simulink model "twolvl_test"  (Simulink 7.5)
settings: Solver=ode45  StartTime=0.0  StopTime=0.5  RelTol=1e-3
undefined symbols (not defined in the file or in its folder): D1, Delta, Ts
libraries: powerlib x18, powerlib_extras x1
settings Model: Creator=IS  LastModifiedBy=IS
settings SolverCC: ZeroCrossAlgorithm=Adaptive

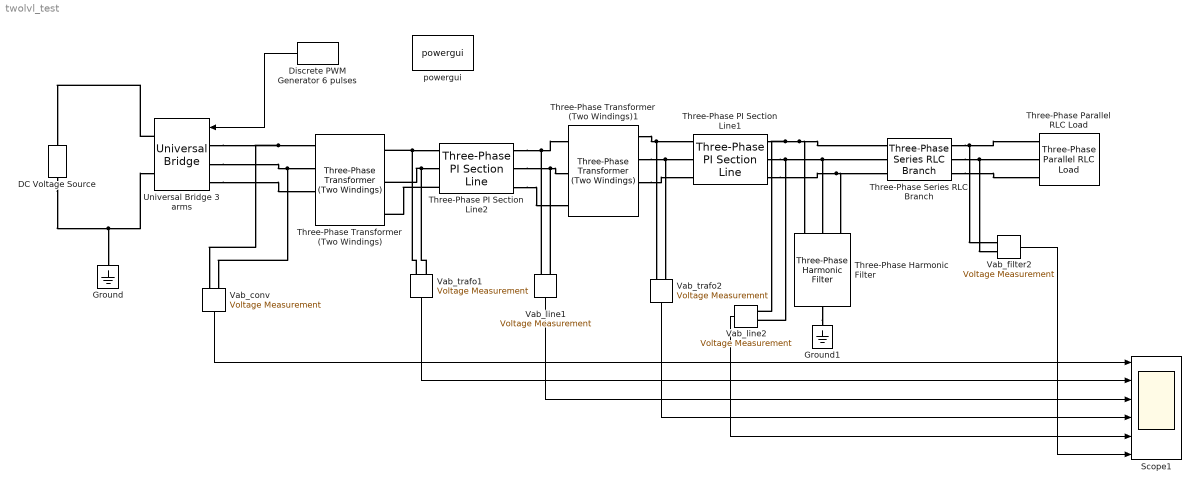
== system twolvl_test ==
  DC Voltage Source : powerlib/Electrical Sources/DC Voltage Source  DialogController=POWERSYS.PowerSysDialog  SystemSampleTime=-1  Amplitude=10e3  Measurements=None
  Discrete PWM Generator 6 pulses : powerlib_extras/Discrete  Control Blocks/Discrete PWM Generator  DialogController=POWERSYS.PowerSysDialog  SystemSampleTime=-1  GeneratorMode="3-arm  bridge (6 pulses)"  Fc=1080  Ts=Ts  Internal=on  mIndex=0.85  Freq=60  Phase=0
  Ground : powerlib/Elements/Ground  DialogController=POWERSYS.PowerSysDialog  PhysicalDomain=powersysdomain  SubClassName=unknown  LeftPortType=p1  RightPortType=p1  LConnTagsString=a
  Ground1 : powerlib/Elements/Ground  DialogController=POWERSYS.PowerSysDialog  PhysicalDomain=powersysdomain  SubClassName=unknown  LeftPortType=p1  RightPortType=p1  LConnTagsString=a
  Scope1 : Scope  NumInputPorts=6
      settings: TimeRange=0.5  YMin=-500~-400~-5~-5~-5~-5  YMax=500~500~5~5~5~5  SaveName=psb3phPWM1_str  MaxDataPoints=500000
  Three-Phase Harmonic Filter : powerlib/Elements/Three-Phase Harmonic Filter  DialogController=POWERSYS.PowerSysDialog  PhysicalDomain=powersysdomain  SubClassName=unknown  LeftPortType=p1  RightPortType=p1  LConnTagsString=A|B|C  RConnTagsString=n  FilterType=Double-tuned  FilterConnection=Y (neutral)  ParNom=[106e3 50]  Qc=100e6  Fr=[5*50]  Frd=[11*50 13*50]  Q=16  Measurements=None
      settings: AttributesFormatString=\n
  Three-Phase PI Section Line1 : powerlib/Elements/Three-Phase PI Section Line  DialogController=POWERSYS.PowerSysDialog  PhysicalDomain=powersysdomain  SubClassName=unknown  LeftPortType=p1  RightPortType=p1  LConnTagsString=a|b|c  RConnTagsString=A|B|C  Frequency=50  Resistances=[ 0.01273 0.3864]  Inductances="[ 0.9337e-3  4.1264e-3]"  Capacitances=[12.74e-9 7.751e-9]  Length=58
  Three-Phase PI Section Line2 : powerlib/Elements/Three-Phase PI Section Line  DialogController=POWERSYS.PowerSysDialog  PhysicalDomain=powersysdomain  SubClassName=unknown  LeftPortType=p1  RightPortType=p1  LConnTagsString=a|b|c  RConnTagsString=A|B|C  Frequency=50  Resistances=[ 0.01273 0.3864]  Inductances="[ 0.9337e-3  4.1264e-3]"  Capacitances=[12.74e-9 7.751e-9]  Length=8
  Three-Phase Parallel RLC Load : powerlib/Elements/Three-Phase Parallel RLC Load  DialogController=POWERSYS.PowerSysDialog  PhysicalDomain=powersysdomain  SubClassName=unknown  LeftPortType=p1  RightPortType=p1  LConnTagsString=A|B|C  Configuration=Y (grounded)  NominalVoltage=106e3  NominalFrequency=50  ActivePower=10e3  InductivePower=100  CapacitivePower=100  Measurements=None
  Three-Phase Series RLC Branch : powerlib/Elements/Three-Phase Series RLC Branch  DialogController=POWERSYS.PowerSysDialog  PhysicalDomain=powersysdomain  SubClassName=unknown  LeftPortType=p1  RightPortType=p1  LConnTagsString=A|B|C  RConnTagsString=A|B|C  BranchType=L  Resistance=1.0  Inductance=1e-3  Capacitance=1.0  Measurements=None
  Three-Phase Transformer (Two Windings) : powerlib/Elements/Three-Phase Transformer (Two Windings)  DialogController=POWERSYS.PowerSysDialog  SystemSampleTime=-1  Winding1Connection=Yn  UNITS=pu  NominalPower=[ 250e6 , 50 ]  Winding1=[ 7e3 , 0.002 , 0.08 ]  Winding2Connection=Delta (D1)  Winding2=[ 23e3 , 0.002 , 0.08 ]  SetSaturation=off  Rm=500  Lm=500  Saturation=[ 0,0 ; 0.0024,1.2 ; 1.0,1.52 ]  Hysteresis=off  DataFile='hysteresis'  SetInitialFlux=off  InitialFluxes=[ 0.8 , -0.8 , 0.7 ]  Measurements=None  MoreParameters=off  BreakLoop=off  DataType=off  TransfoNumber=1
  Three-Phase Transformer (Two Windings)1 : powerlib/Elements/Three-Phase Transformer (Two Windings)  DialogController=POWERSYS.PowerSysDialog  SystemSampleTime=-1  Winding1Connection=Delta (D1)  UNITS=pu  NominalPower=[ 250e6 , 60 ]  Winding1=[ 23e3 , 0.002 , 0.08 ]  Winding2Connection=Yn  Winding2=[ 106e3 , 0.002 , 0.08 ]  SetSaturation=off  Rm=500  Lm=500  Saturation=[ 0,0 ; 0.0024,1.2 ; 1.0,1.52 ]  Hysteresis=off  DataFile='hysteresis'  SetInitialFlux=off  InitialFluxes=[ 0.8 , -0.8 , 0.7 ]  Measurements=None  MoreParameters=off  BreakLoop=off  DataType=off  TransfoNumber=1
  Universal Bridge 3 arms : powerlib/Power Electronics/Universal Bridge  DialogController=POWERSYS.PowerSysDialog  SystemSampleTime=-1  Arms=3  SnubberResistance=10000  SnubberCapacitance=inf  Device=IGBT / Diodes  Ron=1e-4  Lon=0  ForwardVoltages="[  1  1  ]"  ForwardVoltage=.8  GTOparameters=[ 10e-6 , 20e-6 ]  IGBTparameters=[ 1e-6 , 2e-6 ]  Measurements=None  Measurements_2=None  converterType=Rectifier
  Vab_conv : powerlib/Measurements/Voltage Measurement  Tag=PoWeRsYsTeMmEaSuReMeNt  DialogController=POWERSYS.PowerSysDialog  SystemSampleTime=-1  PhasorSimulation=off  OutputType=Magnitude  PSBequivalent=0
  Vab_filter2 : powerlib/Measurements/Voltage Measurement  Tag=PoWeRsYsTeMmEaSuReMeNt  DialogController=POWERSYS.PowerSysDialog  SystemSampleTime=-1  PhasorSimulation=off  OutputType=Magnitude  PSBequivalent=0
  Vab_line1 : powerlib/Measurements/Voltage Measurement  Tag=PoWeRsYsTeMmEaSuReMeNt  DialogController=POWERSYS.PowerSysDialog  SystemSampleTime=-1  PhasorSimulation=off  OutputType=Magnitude  PSBequivalent=0
  Vab_line2 : powerlib/Measurements/Voltage Measurement  Tag=PoWeRsYsTeMmEaSuReMeNt  DialogController=POWERSYS.PowerSysDialog  SystemSampleTime=-1  PhasorSimulation=off  OutputType=Magnitude  PSBequivalent=0
  Vab_trafo1 : powerlib/Measurements/Voltage Measurement  Tag=PoWeRsYsTeMmEaSuReMeNt  DialogController=POWERSYS.PowerSysDialog  SystemSampleTime=-1  PhasorSimulation=off  OutputType=Magnitude  PSBequivalent=0
  Vab_trafo2 : powerlib/Measurements/Voltage Measurement  Tag=PoWeRsYsTeMmEaSuReMeNt  DialogController=POWERSYS.PowerSysDialog  SystemSampleTime=-1  PhasorSimulation=off  OutputType=Magnitude  PSBequivalent=0
  powergui : powerlib/powergui  Priority=1  SystemSampleTime=-1  SimulationMode=Continuous  SampleTime=50e-6  frequency=60  SPID=off  DisableSnubberDevices=off  DisableRonSwitches=off  DisableVfSwitches=off  SwTol=0  Interpol=off  frequencyindice=0  echomessages=off  HookPort=off  DisplayEquations=off  FunctionMessages=off  EnableUseOfTLC=off  x0status=blocks  RestoreLinks=warning  ResistiveCurrentMeasurement=off  Ylog=off  Xlog=on  ShowGrid=off  save=off  variable=ZData  structure=psb3phPWM1_str  ZoomFFT=off  StartTime=0.2  cycles=3  DisplayStyle=1  fundamental=50  FreqAxis=on  MaxFrequency=500  frequencyindicesteady=1  display=off  methode=off
  wires:
  Discrete PWM Generator 6 pulses/1 -> Universal Bridge 3 arms/1
  Vab_filter2/1 -> Scope1/6
  Vab_line2/1 -> Scope1/5
  Vab_trafo2/1 -> Scope1/4
  Vab_line1/1 -> Scope1/3
  Vab_trafo1/1 -> Scope1/2
  Vab_conv/1 -> Scope1/1
  connections:
  Universal Bridge 3 arms/RConn1 -- DC Voltage Source/RConn1
  Universal Bridge 3 arms/RConn2 -- DC Voltage Source/LConn1 -- Ground/LConn1
  Universal Bridge 3 arms/LConn1 -- Three-Phase Transformer (Two Windings)/LConn1 -- Vab_conv/LConn1
  Universal Bridge 3 arms/LConn2 -- Three-Phase Transformer (Two Windings)/LConn2 -- Vab_conv/LConn2
  Universal Bridge 3 arms/LConn3 -- Three-Phase Transformer (Two Windings)/LConn3
  Vab_trafo1/LConn1 -- Three-Phase Transformer (Two Windings)/RConn1 -- Three-Phase PI Section Line2/LConn1
  Vab_trafo1/LConn2 -- Three-Phase Transformer (Two Windings)/RConn2 -- Three-Phase PI Section Line2/LConn2
  Three-Phase Transformer (Two Windings)1/RConn1 -- Three-Phase PI Section Line1/LConn1 -- Vab_trafo2/LConn1
  Three-Phase Transformer (Two Windings)1/RConn2 -- Three-Phase PI Section Line1/LConn2 -- Vab_trafo2/LConn2
  Three-Phase Transformer (Two Windings)1/RConn3 -- Three-Phase PI Section Line1/LConn3
  Three-Phase Harmonic Filter/RConn1 -- Ground1/LConn1
  Three-Phase PI Section Line1/RConn1 -- Three-Phase Series RLC Branch/LConn1 -- Three-Phase Harmonic Filter/LConn1 -- Vab_line2/LConn1
  Three-Phase PI Section Line1/RConn2 -- Three-Phase Series RLC Branch/LConn2 -- Three-Phase Harmonic Filter/LConn2 -- Vab_line2/LConn2
  Three-Phase PI Section Line1/RConn3 -- Three-Phase Series RLC Branch/LConn3 -- Three-Phase Harmonic Filter/LConn3
  Three-Phase Series RLC Branch/RConn1 -- Three-Phase Parallel RLC Load/LConn1 -- Vab_filter2/LConn1
  Three-Phase Series RLC Branch/RConn2 -- Three-Phase Parallel RLC Load/LConn2 -- Vab_filter2/LConn2
  Three-Phase Series RLC Branch/RConn3 -- Three-Phase Parallel RLC Load/LConn3
  Vab_line1/LConn1 -- Three-Phase Transformer (Two Windings)1/LConn1 -- Three-Phase PI Section Line2/RConn1
  Vab_line1/LConn2 -- Three-Phase Transformer (Two Windings)1/LConn2 -- Three-Phase PI Section Line2/RConn2
  Three-Phase PI Section Line2/RConn3 -- Three-Phase Transformer (Two Windings)1/LConn3
  Three-Phase PI Section Line2/LConn3 -- Three-Phase Transformer (Two Windings)/RConn3
